simulink model "Simulation"  (R2023b)
settings: Solver=ode4  StartTime=0.0  StopTime=Te  FixedStep=Ts/20  RelTol=1e-3
undefined symbols (not defined in the file): driving, EgoCar1_params, MPC, mv0, targetSpeed, Ts, waypoints, Weights, x0
libraries: drivingscenarioandsensors x7, robotcorelib x2, mpclib x1, trackingutilitieslib x1, sensorinslib x1, drivinglib x1
settings Model: NumberOfSteps=10  SnapshotBufferSize=1000  SnapshotInterval=100  Creator=Victor  LastModifiedBy=Administrator
settings SolverCC: ZeroCrossAlgorithm=Adaptive
settings DebuggingCC: IgnoredZcDiagnostic=none
settings RTWCC: Toolchain=MinGW64 | CMake/gmake (64-bit Windows)  BuildConfiguration=Release

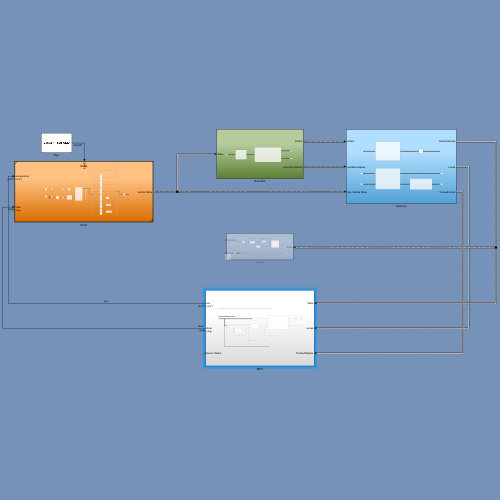
[thumbnail: Simulink's stored preview of the top-level diagram]
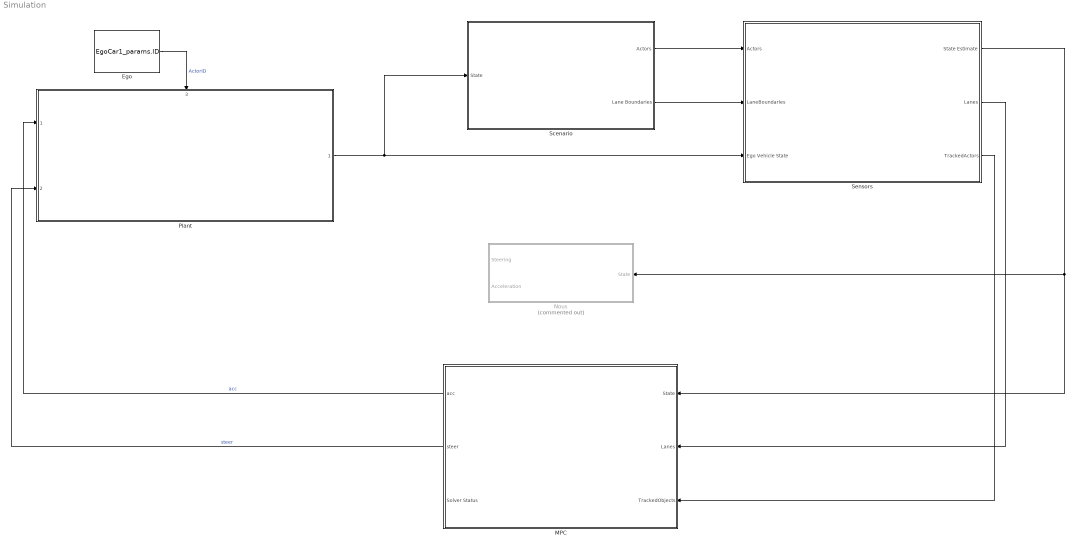
== system Simulation ==
  Ego : Constant  Value=EgoCar1_params.ID
  MPC : Subsystem
  Nous : Subsystem  Commented=on  TreatAsAtomicUnit=on  SystemSampleTime=Ts
  Plant : Subsystem  TreatAsAtomicUnit=on  ReferencedSubsystem=Soma
      settings: MinAlgLoopOccurrences=on  PortSchema="{\"entries\":[{\"content\":{\"sides\":[{\"content\":{\"connectorIds\":[\"In1\",\"In2\"]},\"type\":\"ConnectorPlacement.EquallySpacedRectSide\",\"uuid\":\"82aec969-d257-4f7e-b4fb-71e676d562f3\"},{\"content\":{\"connectorIds\":[\"Out1\"],\"side\":\"RIGHT\"},\"type\":\"ConnectorPlacement.EquallySpacedRectSide\",\"uuid\":\"f71f46c3-49a0-4a72-a46c-a54026d0f764\"},{\"content\":{\"connectorIds\":[\"In3\"],\"side\":\"TOP\"},\"type\":\"ConnectorPlacement.EquallySpacedRectSide\",\"uuid\":\"bd658373-d3b1-4890-887d-293a026755f3\"}]},\"type\":\"ConnectorPlacement.EquallySpacedConnector\",\"uuid\":\"711f2f1f-5cb1-45fa-aff1-e378691897a1\"}],\"packageUris\":[\"http://schema.mathworks.com/mf0/Connector/R2020b\"],\"version\":\"1.0\"}"
  Scenario : Subsystem  SystemSampleTime=Ts
  Sensors : Subsystem
  wires:
  Sensors/1(State Estimate) -> Nous/1(State), MPC/1(State)
  MPC/1(acc) -> Plant/1  "acc"
  MPC/2(steer) -> Plant/2  "steer"
  Ego/1 -> Plant/3  "ActorID"
  Plant/1 -> Scenario/1(State), Sensors/3(Ego Vehicle State)
  Scenario/1(Actors) -> Sensors/1(Actors)
  Scenario/2(Lane Boundaries) -> Sensors/2(LaneBoundaries)
  Sensors/2(Lanes) -> MPC/2(Lanes)
  Sensors/3(TrackedActors) -> MPC/3(TrackedObjects)

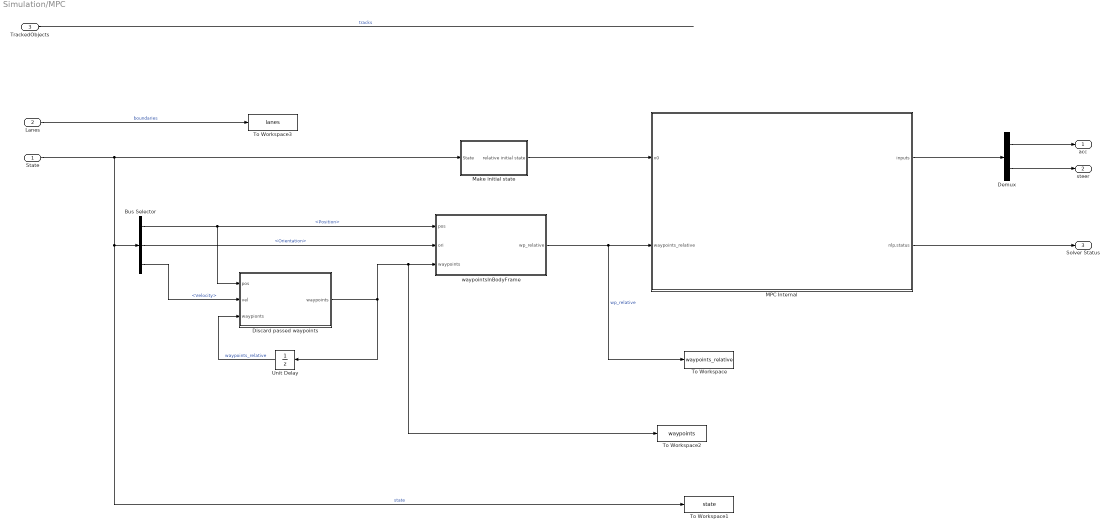
== system Simulation/MPC ==
  State : Inport  OutDataTypeStr=Bus: BusEgoVehicleState  SampleTime=Ts
  Lanes : Inport  Port=2  SampleTime=Ts
  TrackedObjects : Inport  Port=3  SampleTime=Ts
  Bus Selector : BusSelector  OutputSignals=Position,Orientation,Velocity
  Demux : Demux  Outputs=2
  Discard passed waypoints : MATLAB Function  TreatAsAtomicUnit=on
  MPC Internal : Subsystem
  Make initial state : Subsystem
  To Workspace : ToWorkspace  VariableName=waypoints_relative  SaveFormat=Timeseries  SampleTime=-1
  To Workspace1 : ToWorkspace  VariableName=state  SaveFormat=Timeseries  SampleTime=-1
  To Workspace2 : ToWorkspace  VariableName=waypoints  SaveFormat=Timeseries  SampleTime=-1
  To Workspace3 : ToWorkspace  VariableName=lanes  SaveFormat=Timeseries  SampleTime=-1
  Unit Delay : UnitDelay  InitialCondition=waypoints  SampleTime=Ts  HasFrameUpgradeWarning=on
  waypointsInBodyFrame : MATLAB Function  TreatAsAtomicUnit=on
  acc : Outport  Unit=m/s^2  PortDimensions=1  SampleTime=Ts
  steer : Outport  Port=2  Unit=deg  PortDimensions=1  SampleTime=Ts
  Solver Status : Outport  Port=3
  wires:
  State/1 -> Make initial state/1(State), To Workspace1/1, Bus Selector/1  "state"
  Bus Selector/1 -> Discard passed waypoints/1(pos), waypointsInBodyFrame/1(pos)  "<Position>"
  Bus Selector/3 -> Discard passed waypoints/2(vel)  "<Velocity>"
  TrackedObjects/1 -> ?  "tracks"
  waypointsInBodyFrame/1(wp_relative) -> To Workspace/1, MPC Internal/2(waypoints_relative)  "wp_relative"
  Lanes/1 -> To Workspace3/1  "boundaries"
  Demux/1 -> acc/1
  Demux/2 -> steer/1
  MPC Internal/2(nlp.status) -> Solver Status/1
  MPC Internal/1(inputs) -> Demux/1
  Make initial state/1(relative initial state) -> MPC Internal/1(x0)
  Discard passed waypoints/1(waypoints) -> Unit Delay/1, To Workspace2/1, waypointsInBodyFrame/3(waypoints)
  Bus Selector/2 -> waypointsInBodyFrame/2(ori)  "<Orientation>"
  Unit Delay/1 -> Discard passed waypoints/3(waypionts)  "waypoints_relative"

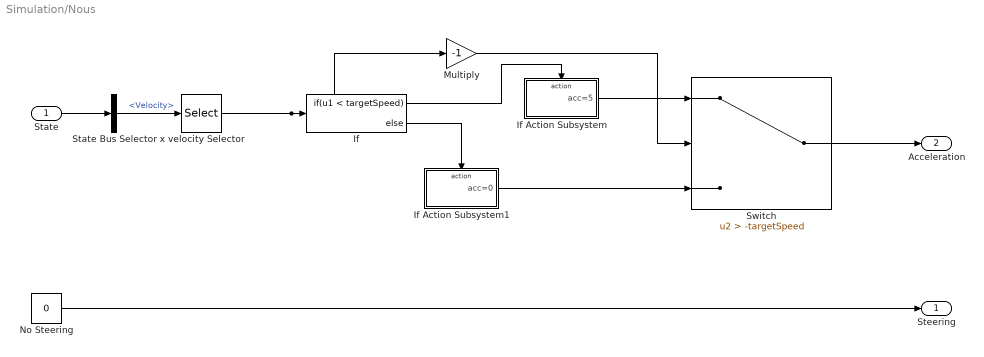
== system Simulation/Nous ==
  State : Inport  SampleTime=Ts
  If : If  IfExpression=u1 < targetSpeed
  If Action Subsystem : Subsystem  TreatAsAtomicUnit=on
  If Action Subsystem1 : Subsystem  TreatAsAtomicUnit=on
  Multiply : Gain  Gain=-1
  No Steering : Constant  Value=0  SampleTime=Ts
  State Bus Selector : BusSelector  OutputSignals=Velocity
  Switch : Switch  Criteria=u2 > Threshold  Threshold=-targetSpeed  SaturateOnIntegerOverflow=off  InputSameDT=off
  x velocity Selector : Selector  InputPortWidth=3  IndexOptions=Index vector (dialog)  Indices=[1]  OutputSizes=1
  Steering : Outport  Unit=deg  SampleTime=Ts
  Acceleration : Outport  Port=2  Unit=m/s^2  SampleTime=Ts
  wires:
  Switch/1 -> Acceleration/1
  If Action Subsystem/1(acc=5) -> Switch/1
  If/1 -> If Action Subsystem/Action
  State/1 -> State Bus Selector/1
  x velocity Selector/1 -> Multiply/1, If/1
  If Action Subsystem1/1(acc=0) -> Switch/3
  No Steering/1 -> Steering/1
  Multiply/1 -> Switch/2
  State Bus Selector/1 -> x velocity Selector/1  "<Velocity>"
  If/2 -> If Action Subsystem1/Action

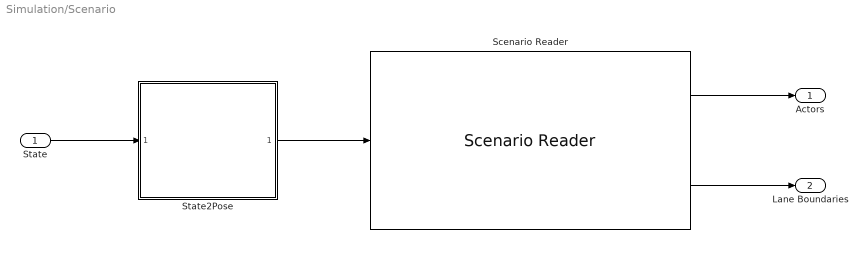
== system Simulation/Scenario ==
  State : Inport
  " State2Pose" : Subsystem  TreatAsAtomicUnit=on  ReferencedSubsystem=State2Pose
  Scenario Reader : drivingscenarioandsensors/Scenario Reader  ScenarioSource=From file  ScenarioFileName=C:\Users\Administrator\Projects\RNNMPC\Scenarios\StraightRoad_Challenge.mat  ScenarioVariableName=Scenario  OutputCoordinateSystem=Vehicle coordinates  EgoVehicleSource=Input port  EgoVehicleActorID=1  OrientVehiclesOnRoad=on  OutputEgoVehiclePose=off  OutputEgoVehicleState=on  SampleTime=Ts  LaneBoundaryOutput=All lane boundaries  LaneBoundaryDistance=linspace(0, 50, 51)  LaneBoundaryLocation=Center of lane markings  BusNameSource=Auto  BusName=BusActors  BusNumActorsSource=Scenario  BusNumActors=32  BusName2Source=Auto  BusName2=BusLaneBoundaries  BusNumLaneBoundariesSource=Scenario  BusNumLaneBoundaries=10  BusName3Source=Auto  BusName3=BusEgoActor  BusName4Source=Auto  BusName4=BusEgoState  ShowCoordinateLabels=on  SimulateUsing=Code generation
  Actors : Outport
  Lane Boundaries : Outport  Port=2
  wires:
  Scenario Reader/1 -> Actors/1
  State/1 -> " State2Pose"/1
  Scenario Reader/2 -> Lane Boundaries/1
  " State2Pose"/1 -> Scenario Reader/1

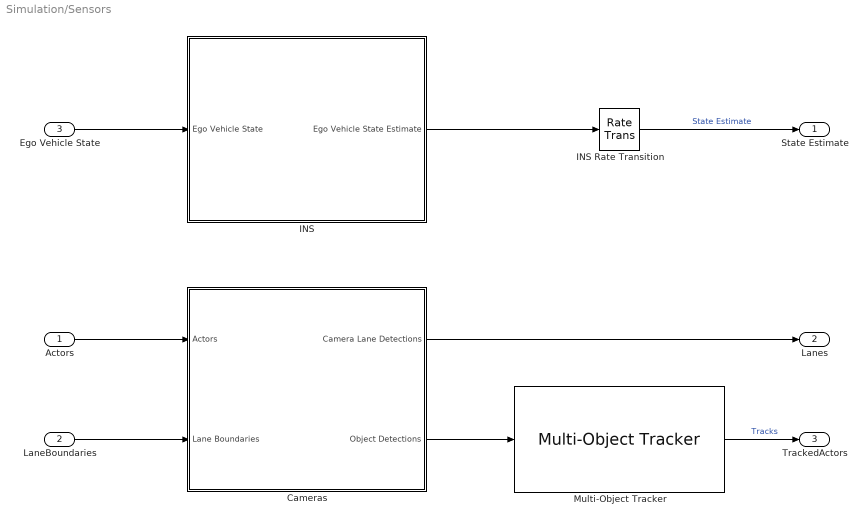
== system Simulation/Sensors ==
  Actors : Inport
  LaneBoundaries : Inport  Port=2
  Ego Vehicle State : Inport  Port=3  OutDataTypeStr=Bus: BusEgoVehicleState
  Cameras : Subsystem
  INS : Subsystem  TreatAsAtomicUnit=on  SystemSampleTime=Ts
  INS Rate Transition : RateTransition  OutPortSampleTime=Ts
  Multi-Object Tracker : drivinglib/Multi-Object Tracker  TrackerIndex=uint32( 0 )  FilterInitializationFcn=initcvekf  AssignmentThreshold=50  ConfirmationThreshold=[ 2, 3 ]  DeletionThreshold=[5,5]  MaxNumTracks=6  MaxNumSensors=8  OOSMHandling=Terminate  StateParametersSimulink=struct  HasStateParametersInput=off  TimeInputSource=Auto  HasCostMatrixInput=off  HasDetectableTrackIDsInput=off  BusNameSource=Auto  BusName=BusMultiObjectTracker1  TentativeTracksOutputPort=off  AllTracksOutputPort=off  SimulateUsing=Interpreted execution
  State Estimate : Outport
  Lanes : Outport  Port=2  SampleTime=Ts
  TrackedActors : Outport  Port=3  SampleTime=Ts
  wires:
  Ego Vehicle State/1 -> INS/1(Ego Vehicle State)
  INS Rate Transition/1 -> State Estimate/1  "State Estimate"
  INS/1(Ego Vehicle State Estimate) -> INS Rate Transition/1
  Multi-Object Tracker/1 -> TrackedActors/1  "Tracks"
  Actors/1 -> Cameras/1(Actors)
  LaneBoundaries/1 -> Cameras/2(Lane Boundaries)
  Cameras/1(Camera Lane Detections) -> Lanes/1
  Cameras/2(Object Detections) -> Multi-Object Tracker/1

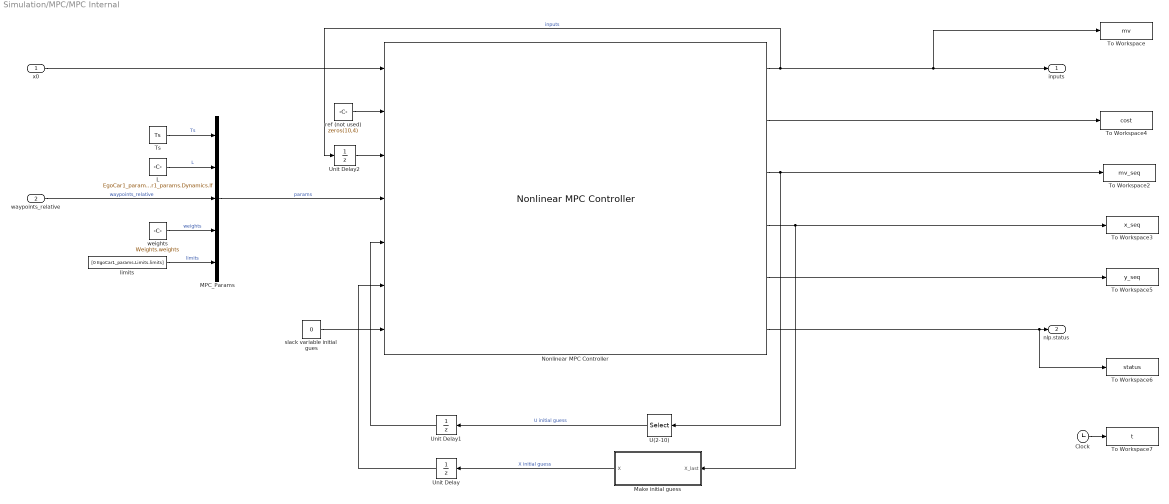
== system Simulation/MPC/MPC Internal ==
  x0 : Inport
  waypoints_relative : Inport  Port=2
  Clock : Clock
  L : Constant  Value=EgoCar1_params.Dynamics.lr+EgoCar1_params.Dynamics.lf  SampleTime=Ts
  MPC_Params : BusCreator  Inputs=5  OutDataTypeStr=Bus: BusParams  NonVirtualBus=on
      settings: InheritFromInputs=off
  Make initial guess : MATLAB Function  TreatAsAtomicUnit=on
  Nonlinear MPC Controller : mpclib/Nonlinear MPC Controller  nlmpcobj=MPC  UseObjectTs=on  UseMEX=off  mexname=nlmpc_MEX  md_enabled=off  mvtarget_enabled=off  param_enabled=on  cost_enabled=on  mvseq_enabled=on  stateseq_enabled=on  ovseq_enabled=on  slack_enabled=off  status_enabled=on  ov_min=off  ov_max=off  mv_min=off  mv_max=off  mvrate_min=off  mvrate_max=off  state_min=off  state_max=off  ov_weight=off  mv_weight=off  mvrate_weight=off  ecr_weight=off  nlp_initialize=on
  To Workspace : ToWorkspace  VariableName=mv  SaveFormat=Timeseries  SampleTime=-1
  To Workspace2 : ToWorkspace  VariableName=mv_seq  SaveFormat=Timeseries  SampleTime=-1
  To Workspace3 : ToWorkspace  VariableName=x_seq  SaveFormat=Timeseries  SampleTime=-1
  To Workspace4 : ToWorkspace  VariableName=cost  SaveFormat=Timeseries  SampleTime=-1
  To Workspace5 : ToWorkspace  VariableName=y_seq  SaveFormat=Timeseries  SampleTime=-1
  To Workspace6 : ToWorkspace  VariableName=status  SaveFormat=Timeseries  SampleTime=-1
  To Workspace7 : ToWorkspace  VariableName=t  SaveFormat=Timeseries  SampleTime=-1
  Ts : Constant  Value=Ts  SampleTime=Ts
  U(2-10) : Selector  NumberOfDimensions=2  InputPortWidth=3  IndexOptions=Index vector (dialog),Index vector (dialog)  Indices=[2:MPC.PredictionHorizon+1],[1:2]  OutputSizes=1,1
  Unit Delay : UnitDelay  InitialCondition=repmat(x0',10,1)  SampleTime=Ts  HasFrameUpgradeWarning=on
  Unit Delay1 : UnitDelay  InitialCondition=repmat(mv0',10,1)  SampleTime=Ts  HasFrameUpgradeWarning=on
  Unit Delay2 : UnitDelay  SampleTime=Ts  HasFrameUpgradeWarning=on
  limits : FromWorkspace  VariableName=[0 EgoCar1_params.Limits.limits]  SampleTime=Ts  Interpolate=off  OutputAfterFinalValue=Holding final value
  ref (not used) : Constant  Value=zeros(10,4)
  slack variable initial gues : Constant  Value=0
  weights : Constant  Value=Weights.weights  SampleTime=Ts
  inputs : Outport
  nlp.status : Outport  Port=2
  wires:
  Nonlinear MPC Controller/5 -> To Workspace5/1
  Nonlinear MPC Controller/1 -> To Workspace/1, inputs/1, Unit Delay2/1  "inputs"
  Nonlinear MPC Controller/6 -> To Workspace6/1, nlp.status/1
  Unit Delay1/1 -> Nonlinear MPC Controller/5
  slack variable initial gues/1 -> Nonlinear MPC Controller/7
  ref (not used)/1 -> Nonlinear MPC Controller/2
  Nonlinear MPC Controller/3 -> To Workspace2/1, U(2-10)/1
  U(2-10)/1 -> Unit Delay1/1  "U initial guess"
  Unit Delay/1 -> Nonlinear MPC Controller/6
  Unit Delay2/1 -> Nonlinear MPC Controller/3
  Nonlinear MPC Controller/2 -> To Workspace4/1
  waypoints_relative/1 -> MPC_Params/3  "waypoints_relative"
  x0/1 -> Nonlinear MPC Controller/1
  L/1 -> MPC_Params/2  "L"
  Ts/1 -> MPC_Params/1  "Ts"
  weights/1 -> MPC_Params/4  "weights"
  MPC_Params/1 -> Nonlinear MPC Controller/4  "params"
  limits/1 -> MPC_Params/5  "limits"
  Make initial guess/1(X) -> Unit Delay/1  "X initial guess"
  Nonlinear MPC Controller/4 -> Make initial guess/1(X_last), To Workspace3/1
  Clock/1 -> To Workspace7/1

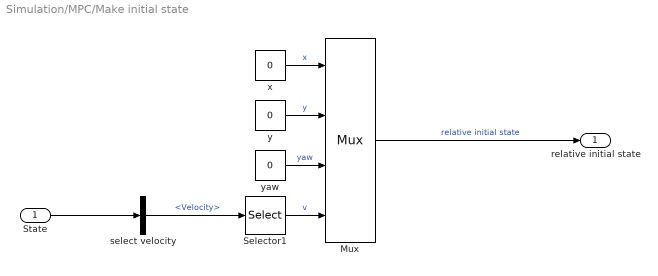
== system Simulation/MPC/Make initial state ==
  State : Inport
  Mux : Mux
      settings: DisplayOption=signals
  Selector1 : Selector  InputPortWidth=3  IndexOptions=Index vector (dialog)  Indices=1  OutputSizes=1
  select velocity : BusSelector  OutputSignals=Velocity
  x : Constant  Value=0
  y : Constant  Value=0
  yaw : Constant  Value=0
  relative initial state : Outport
  wires:
  y/1 -> Mux/2  "y"
  Mux/1 -> relative initial state/1  "relative initial state"
  x/1 -> Mux/1  "x"
  yaw/1 -> Mux/3  "yaw"
  Selector1/1 -> Mux/4  "v"
  select velocity/1 -> Selector1/1  "<Velocity>"
  State/1 -> select velocity/1

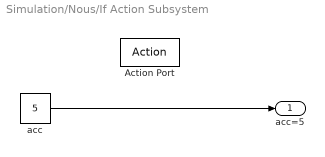
== system Simulation/Nous/If Action Subsystem ==
  Action Port : ActionPort  ActionPortLabel=if(u1 < targetSpeed)
  acc : Constant  Value=5
  acc=5 : Outport
  wires:
  acc/1 -> acc=5/1

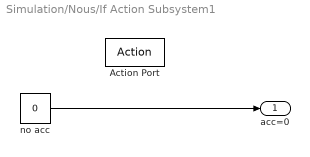
== system Simulation/Nous/If Action Subsystem1 ==
  Action Port : ActionPort  ActionPortLabel=else
  no acc : Constant  Value=0
  acc=0 : Outport
  wires:
  no acc/1 -> acc=0/1

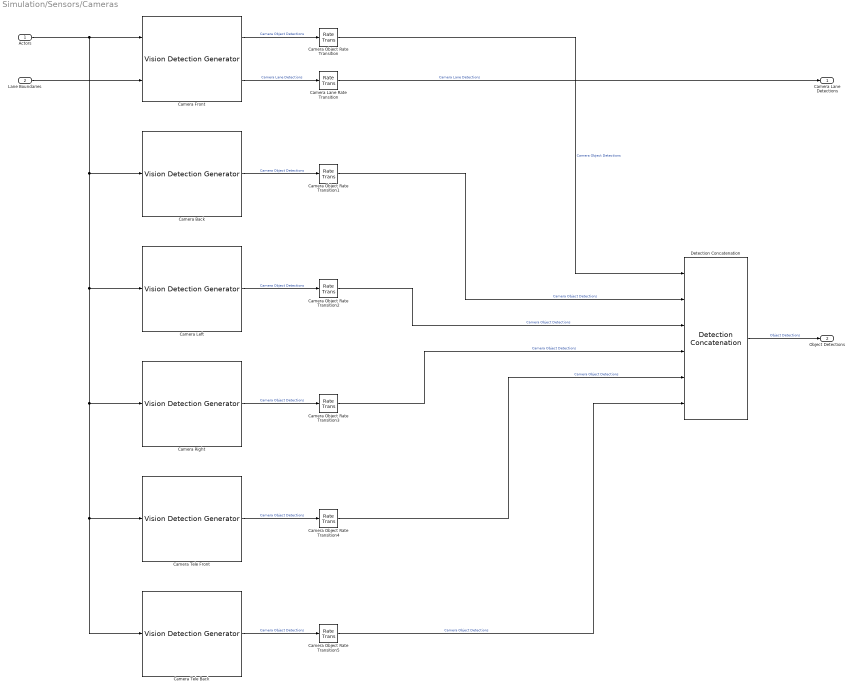
== system Simulation/Sensors/Cameras ==
  Actors : Inport
  Lane Boundaries : Inport  Port=2
  Camera Back : drivingscenarioandsensors/Vision Detection Generator  SensorIndex=3  DetectorOutput=Objects only  UpdateInterval=Ts  LaneUpdateInterval=Ts  SensorLocation=[ 1.9, 0 ]  Height=1.1  Yaw=EgoCar1_params.Sensors.cameras(2).Direction  Pitch=1  Roll=0  BusNameSource=Auto  BusName=BusObjectDetections  BusName2Source=Auto  BusName2=BusLaneDetections  MaxNumDetectionsSource=Property  MaxNumDetections=6  MaxNumLanesSource=Property  MaxNumLanes=30  DetectionCoordinates=Ego Cartesian  SimulateUsing=Code generation  MaxRange=EgoCar1_params.Sensors.cameras(2).Range_Max  BoundingBoxAccuracy=5  ProcessNoiseIntensity=5  MaxSpeed=100  MaxAllowedOcclusion=0.5  MinObjectImageSize=[ 15, 15 ]  DetectionProbability=0.9  FalsePositivesPerImage=0  MinLaneImageSize=[ 20, 3 ]  LaneBoundaryAccuracy=3  HasNoise=off  InitialSeedSource=Repeatable  InitialSeed=0  UsedSeed=driving.internal.SimulinkUtilities.seedManager(gcb)  ActorProfilesSource=From Scenario Reader block  ActorProfilesParameters=driving.internal.ActorProfilesParameters  ActorProfilesExpression=struct( 'ClassID', 0, 'Length', 4.7, 'Width', 1.8, 'Height', 1.4, 'OriginOffset', [ -1.35, 0, 0 ] )  Intrinsics=driving.internal.cameraIntrinsics(FocalLength=[ EgoCar1_params.Sensors.cameras(2).FocalLength_X, EgoCar1_params.Sensors.cameras(2).FocalLength_Y],PrincipalPoint=[ EgoCar1_params.Sensors.cameras(2).OpticalCenter_X, EgoCar1_params.Sensors.cameras(2).OpticalCenter_Y],ImageSize=[ EgoCar1_params.Sensors.cameras(2).Image_Height, EgoCar1_params.Sensors.cameras(2).Image_Width])
  Camera Front : drivingscenarioandsensors/Vision Detection Generator  SensorIndex=2  DetectorOutput=Lanes and objects  UpdateInterval=Ts  LaneUpdateInterval=Ts  SensorLocation=[ 1.9, 0 ]  Height=1.1  Yaw=EgoCar1_params.Sensors.cameras(1).Direction  Pitch=1  Roll=0  BusNameSource=Auto  BusName=BusObjectDetections  BusName2Source=Auto  BusName2=BusLaneDetections  MaxNumDetectionsSource=Property  MaxNumDetections=6  MaxNumLanesSource=Property  MaxNumLanes=12  DetectionCoordinates=Ego Cartesian  SimulateUsing=Code generation  MaxRange=EgoCar1_params.Sensors.cameras(1).Range_Max  BoundingBoxAccuracy=5  ProcessNoiseIntensity=5  MaxSpeed=100  MaxAllowedOcclusion=0.5  MinObjectImageSize=[ 15, 15 ]  DetectionProbability=0.9  FalsePositivesPerImage=0  MinLaneImageSize=[10, 3]  LaneBoundaryAccuracy=3  HasNoise=off  InitialSeedSource=Repeatable  InitialSeed=0  UsedSeed=driving.internal.SimulinkUtilities.seedManager(gcb)  ActorProfilesSource=From Scenario Reader block  ActorProfilesParameters=driving.internal.ActorProfilesParameters  ActorProfilesExpression=struct( 'ClassID', 0, 'Length', 4.7, 'Width', 1.8, 'Height', 1.4, 'OriginOffset', [ -1.35, 0, 0 ] )  Intrinsics=driving.internal.cameraIntrinsics(FocalLength=[ EgoCar1_params.Sensors.cameras(1).FocalLength_X, EgoCar1_params.Sensors.cameras(1).FocalLength_Y],PrincipalPoint=[ EgoCar1_params.Sensors.cameras(1).OpticalCenter_X, EgoCar1_params.Sensors.cameras(1).OpticalCenter_Y],ImageSize=[ EgoCar1_params.Sensors.cameras(1).Image_Height, EgoCar1_params.Sensors.cameras(1).Image_Width])
  Camera Lane Rate Transition : RateTransition  OutPortSampleTime=Ts
  Camera Left : drivingscenarioandsensors/Vision Detection Generator  SensorIndex=4  DetectorOutput=Objects only  UpdateInterval=Ts  LaneUpdateInterval=Ts  SensorLocation=[ 1.9, 0 ]  Height=1.1  Yaw=EgoCar1_params.Sensors.cameras(3).Direction  Pitch=1  Roll=0  BusNameSource=Auto  BusName=BusObjectDetections  BusName2Source=Auto  BusName2=BusLaneDetections  MaxNumDetectionsSource=Property  MaxNumDetections=6  MaxNumLanesSource=Property  MaxNumLanes=30  DetectionCoordinates=Ego Cartesian  SimulateUsing=Code generation  MaxRange=EgoCar1_params.Sensors.cameras(3).Range_Max  BoundingBoxAccuracy=5  ProcessNoiseIntensity=5  MaxSpeed=100  MaxAllowedOcclusion=0.5  MinObjectImageSize=[ 15, 15 ]  DetectionProbability=0.9  FalsePositivesPerImage=0  MinLaneImageSize=[ 20, 3 ]  LaneBoundaryAccuracy=3  HasNoise=off  InitialSeedSource=Repeatable  InitialSeed=0  UsedSeed=driving.internal.SimulinkUtilities.seedManager(gcb)  ActorProfilesSource=From Scenario Reader block  ActorProfilesParameters=driving.internal.ActorProfilesParameters  ActorProfilesExpression=struct( 'ClassID', 0, 'Length', 4.7, 'Width', 1.8, 'Height', 1.4, 'OriginOffset', [ -1.35, 0, 0 ] )  Intrinsics=driving.internal.cameraIntrinsics(FocalLength=[ EgoCar1_params.Sensors.cameras(3).FocalLength_X, EgoCar1_params.Sensors.cameras(3).FocalLength_Y],PrincipalPoint=[ EgoCar1_params.Sensors.cameras(3).OpticalCenter_X, EgoCar1_params.Sensors.cameras(3).OpticalCenter_Y],ImageSize=[ EgoCar1_params.Sensors.cameras(3).Image_Height, EgoCar1_params.Sensors.cameras(3).Image_Width])
  Camera Object Rate Transition{,1..5} (6 alike) : RateTransition  OutPortSampleTime=Ts
  Camera Right : drivingscenarioandsensors/Vision Detection Generator  SensorIndex=5  DetectorOutput=Objects only  UpdateInterval=Ts  LaneUpdateInterval=Ts  SensorLocation=[ 1.9, 0 ]  Height=1.1  Yaw=EgoCar1_params.Sensors.cameras(4).Direction  Pitch=1  Roll=0  BusNameSource=Auto  BusName=BusObjectDetections  BusName2Source=Auto  BusName2=BusLaneDetections  MaxNumDetectionsSource=Property  MaxNumDetections=6  MaxNumLanesSource=Property  MaxNumLanes=30  DetectionCoordinates=Ego Cartesian  SimulateUsing=Code generation  MaxRange=EgoCar1_params.Sensors.cameras(4).Range_Max  BoundingBoxAccuracy=5  ProcessNoiseIntensity=5  MaxSpeed=100  MaxAllowedOcclusion=0.5  MinObjectImageSize=[ 15, 15 ]  DetectionProbability=0.9  FalsePositivesPerImage=0  MinLaneImageSize=[ 20, 3 ]  LaneBoundaryAccuracy=3  HasNoise=off  InitialSeedSource=Repeatable  InitialSeed=0  UsedSeed=driving.internal.SimulinkUtilities.seedManager(gcb)  ActorProfilesSource=From Scenario Reader block  ActorProfilesParameters=driving.internal.ActorProfilesParameters  ActorProfilesExpression=struct( 'ClassID', 0, 'Length', 4.7, 'Width', 1.8, 'Height', 1.4, 'OriginOffset', [ -1.35, 0, 0 ] )  Intrinsics=driving.internal.cameraIntrinsics(FocalLength=[ EgoCar1_params.Sensors.cameras(4).FocalLength_X, EgoCar1_params.Sensors.cameras(4).FocalLength_Y],PrincipalPoint=[ EgoCar1_params.Sensors.cameras(4).OpticalCenter_X, EgoCar1_params.Sensors.cameras(4).OpticalCenter_Y],ImageSize=[ EgoCar1_params.Sensors.cameras(4).Image_Height, EgoCar1_params.Sensors.cameras(4).Image_Width])
  Camera Tele Back : drivingscenarioandsensors/Vision Detection Generator  SensorIndex=7  DetectorOutput=Objects only  UpdateInterval=Ts  LaneUpdateInterval=Ts  SensorLocation=[ 1.9, 0 ]  Height=1.1  Yaw=EgoCar1_params.Sensors.cameras(6).Direction  Pitch=1  Roll=0  BusNameSource=Auto  BusName=BusObjectDetections  BusName2Source=Auto  BusName2=BusLaneDetections  MaxNumDetectionsSource=Property  MaxNumDetections=6  MaxNumLanesSource=Property  MaxNumLanes=30  DetectionCoordinates=Ego Cartesian  SimulateUsing=Code generation  MaxRange=EgoCar1_params.Sensors.cameras(6).Range_Max  BoundingBoxAccuracy=5  ProcessNoiseIntensity=5  MaxSpeed=100  MaxAllowedOcclusion=0.5  MinObjectImageSize=[ 15, 15 ]  DetectionProbability=0.9  FalsePositivesPerImage=0  MinLaneImageSize=[10, 3]  LaneBoundaryAccuracy=3  HasNoise=off  InitialSeedSource=Repeatable  InitialSeed=0  UsedSeed=driving.internal.SimulinkUtilities.seedManager(gcb)  ActorProfilesSource=From Scenario Reader block  ActorProfilesParameters=driving.internal.ActorProfilesParameters  ActorProfilesExpression=struct( 'ClassID', 0, 'Length', 4.7, 'Width', 1.8, 'Height', 1.4, 'OriginOffset', [ -1.35, 0, 0 ] )  Intrinsics=driving.internal.cameraIntrinsics(FocalLength=[ EgoCar1_params.Sensors.cameras(6).FocalLength_X, EgoCar1_params.Sensors.cameras(6).FocalLength_Y],ImageSize=[ EgoCar1_params.Sensors.cameras(6).Image_Height, EgoCar1_params.Sensors.cameras(6).Image_Width],PrincipalPoint=[ EgoCar1_params.Sensors.cameras(6).OpticalCenter_X, EgoCar1_params.Sensors.cameras(6).OpticalCenter_Y])
  Camera Tele Front : drivingscenarioandsensors/Vision Detection Generator  SensorIndex=6  DetectorOutput=Objects only  UpdateInterval=Ts  LaneUpdateInterval=Ts  SensorLocation=[ 1.9, 0 ]  Height=1.1  Yaw=EgoCar1_params.Sensors.cameras(5).Direction  Pitch=1  Roll=0  BusNameSource=Auto  BusName=BusObjectDetections  BusName2Source=Auto  BusName2=BusLaneDetections  MaxNumDetectionsSource=Property  MaxNumDetections=6  MaxNumLanesSource=Property  MaxNumLanes=30  DetectionCoordinates=Ego Cartesian  SimulateUsing=Code generation  MaxRange=EgoCar1_params.Sensors.cameras(5).Range_Max  BoundingBoxAccuracy=5  ProcessNoiseIntensity=5  MaxSpeed=100  MaxAllowedOcclusion=0.5  MinObjectImageSize=[ 15, 15 ]  DetectionProbability=0.9  FalsePositivesPerImage=0  MinLaneImageSize=[10, 3]  LaneBoundaryAccuracy=3  HasNoise=off  InitialSeedSource=Repeatable  InitialSeed=0  UsedSeed=driving.internal.SimulinkUtilities.seedManager(gcb)  ActorProfilesSource=From Scenario Reader block  ActorProfilesParameters=driving.internal.ActorProfilesParameters  ActorProfilesExpression=struct( 'ClassID', 0, 'Length', 4.7, 'Width', 1.8, 'Height', 1.4, 'OriginOffset', [ -1.35, 0, 0 ] )  Intrinsics=driving.internal.cameraIntrinsics(FocalLength=[ EgoCar1_params.Sensors.cameras(5).FocalLength_X, EgoCar1_params.Sensors.cameras(5).FocalLength_Y],ImageSize=[ EgoCar1_params.Sensors.cameras(5).Image_Height, EgoCar1_params.Sensors.cameras(5).Image_Width],PrincipalPoint=[ EgoCar1_params.Sensors.cameras(5).OpticalCenter_X, EgoCar1_params.Sensors.cameras(5).OpticalCenter_Y])
  Detection Concatenation : trackingutilitieslib/Detection Concatenation  NumInputs=6  BusNameSource=Auto  BusName=BusDetectionConcatenation1  SimulateUsing=Interpreted execution
  Camera Lane Detections : Outport
  Object Detections : Outport  Port=2
  wires:
  Camera Front/1 -> Camera Object Rate Transition/1  "Camera Object Detections"
  Camera Left/1 -> Camera Object Rate Transition2/1  "Camera Object Detections"
  Camera Lane Rate Transition/1 -> Camera Lane Detections/1  "Camera Lane Detections"
  Camera Right/1 -> Camera Object Rate Transition3/1  "Camera Object Detections"
  Lane Boundaries/1 -> Camera Front/2
  Camera Object Rate Transition/1 -> Detection Concatenation/1  "Camera Object Detections"
  Camera Object Rate Transition1/1 -> Detection Concatenation/2  "Camera Object Detections"
  Detection Concatenation/1 -> Object Detections/1  "Object Detections"
  Camera Front/2 -> Camera Lane Rate Transition/1  "Camera Lane Detections"
  Camera Object Rate Transition3/1 -> Detection Concatenation/4  "Camera Object Detections"
  Camera Object Rate Transition2/1 -> Detection Concatenation/3  "Camera Object Detections"
  Actors/1 -> Camera Tele Back/1, Camera Tele Front/1, Camera Right/1, Camera Left/1, Camera Back/1, Camera Front/1
  Camera Back/1 -> Camera Object Rate Transition1/1  "Camera Object Detections"
  Camera Tele Front/1 -> Camera Object Rate Transition4/1  "Camera Object Detections"
  Camera Object Rate Transition4/1 -> Detection Concatenation/5  "Camera Object Detections"
  Camera Tele Back/1 -> Camera Object Rate Transition5/1  "Camera Object Detections"
  Camera Object Rate Transition5/1 -> Detection Concatenation/6  "Camera Object Detections"

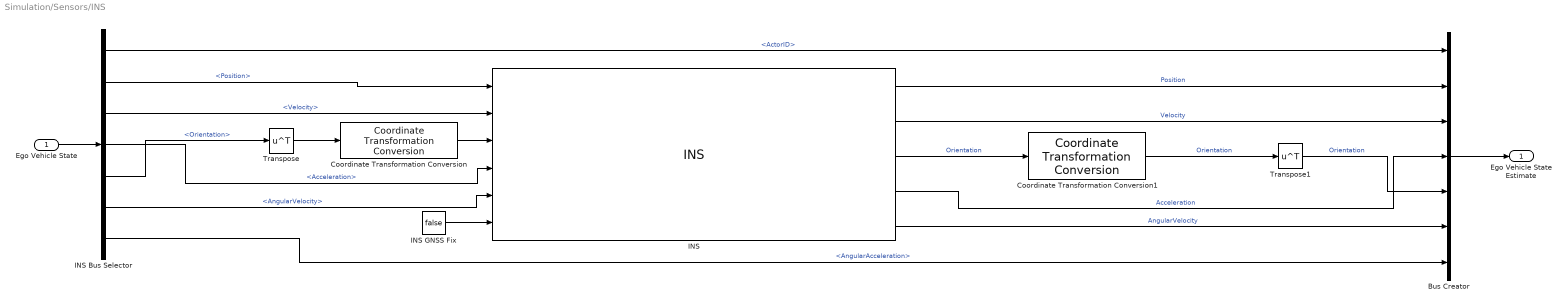
== system Simulation/Sensors/INS ==
  Ego Vehicle State : Inport  OutDataTypeStr=Bus: BusEgoVehicleState
  Bus Creator : BusCreator  Inputs=7  OutDataTypeStr=Bus: BusEgoVehicleState  NonVirtualBus=on
      settings: InheritFromInputs=off
  Coordinate Transformation Conversion : robotcorelib/Coordinate Transformation Conversion  InputRepresentation=Euler Angles  InputEulerSequence=XYZ  ShowTrVecInputPort=on  OutputRepresentation=Rotation Matrix  OutputEulerSequence=ZYX  ShowTrVecOutputPort=on  SimulateUsing=Code generation
      settings: LibrarySourceBlock=navlib/Utilities/Coordinate Transformation Conversion
  Coordinate Transformation Conversion1 : robotcorelib/Coordinate Transformation Conversion  InputRepresentation=Rotation Matrix  InputEulerSequence=ZYX  ShowTrVecInputPort=on  OutputRepresentation=Euler Angles  OutputEulerSequence=XYZ  ShowTrVecOutputPort=on  SimulateUsing=Code generation
      settings: LibrarySourceBlock=navlib/Utilities/Coordinate Transformation Conversion
  INS : sensorinslib/INS  MountingLocation=[0 0 0]  RollAccuracy=EgoCar1_params.Sensors.INS.angleAccuraccy  PitchAccuracy=EgoCar1_params.Sensors.INS.angleAccuraccy  YawAccuracy=EgoCar1_params.Sensors.INS.angleAccuraccy  PositionAccuracy=[EgoCar1_params.Sensors.INS.positionAccuracy EgoCar1_params.Sensors.INS.positionAccuracy EgoCar1_params.Sensors.INS.positionAccuracy]  VelocityAccuracy=EgoCar1_params.Sensors.INS.velocityAccuracy  UseAccelAndAngVel=on  AccelerationAccuracy=0  AngularVelocityAccuracy=0  TimeInput=on  PositionErrorFactor=[0 0 0]  SeedDouble=32  SimulateUsing=Code generation
      settings: LibrarySourceBlock=drivingscenarioandsensors/INS
  INS Bus Selector : BusSelector  OutputSignals=ActorID,Position,Velocity,Acceleration,Orientation,AngularVelocity,AngularAcceleration
  INS GNSS Fix : Constant  Value=false
  Transpose : Math  Operator=transpose
  Transpose1 : Math  Operator=transpose
  Ego Vehicle State Estimate : Outport  OutDataTypeStr=Bus: BusEgoVehicleState
  wires:
  Ego Vehicle State/1 -> INS Bus Selector/1
  INS/2 -> Bus Creator/3  "Velocity"
  Transpose1/1 -> Bus Creator/5  "Orientation"
  INS Bus Selector/3 -> INS/2  "<Velocity>"
  INS/1 -> Bus Creator/2  "Position"
  INS/4 -> Bus Creator/4  "Acceleration"
  Bus Creator/1 -> Ego Vehicle State Estimate/1
  INS/5 -> Bus Creator/6  "AngularVelocity"
  INS GNSS Fix/1 -> INS/6
  Coordinate Transformation Conversion/1 -> INS/3
  INS/3 -> Coordinate Transformation Conversion1/1  "Orientation"
  INS Bus Selector/2 -> INS/1  "<Position>"
  Transpose/1 -> Coordinate Transformation Conversion/1
  Coordinate Transformation Conversion1/1 -> Transpose1/1  "Orientation"
  INS Bus Selector/6 -> INS/5  "<AngularVelocity>"
  INS Bus Selector/1 -> Bus Creator/1  "<ActorID>"
  INS Bus Selector/7 -> Bus Creator/7  "<AngularAcceleration>"
  INS Bus Selector/4 -> INS/4  "<Acceleration>"
  INS Bus Selector/5 -> Transpose/1  "<Orientation>"

== matlab function Simulation/MPC/Discard passed waypoints ==
  data: pos input; waypoints output; vel input; waypionts input
function waypoints = wpts_discard(pos, vel, waypionts)
    waypoints = waypointsTruncation(pos, vel, waypionts);
end

== matlab function Simulation/MPC/MPC Internal/Make initial guess ==
  data: X_last input; X output
function X = makeInitGuess(X_last)
    
    % Discard the state at the previous step
    X=X_last(2:11,:);
    x1=X(1,:);
    
    % Rotation Matrix
    yaw=X(1,3);
    R = [cosd(-yaw), -sind(-yaw); sind(-yaw), cosd(-yaw)];

    for i = 1:size(X,1)
        
        xy=X(i,1:2)';

        % Transformation
        xy=xy-x1(1:2)';
        xy=R * xy;
        X(i,1:2)=xy';

        % Rotation
        X(i,3)=X(i,3)-X(1,3);
    end
end

== matlab function Simulation/MPC/waypointsInBodyFrame ==
  data: pos input; ori input; wp_relative output; waypoints input
function wp_relative = waypointsInBodyFrame(pos, ori, waypoints)
    pos=pos(1:2);
    pos=reshape(pos,2,[]);

    yaw=ori(3);

    wp_relative=NaN(size(waypoints));
    for i=1:size(wp_relative,1)
        wp_relative(i,:) = world2body(pos, yaw, waypoints(i,:)');
    end
end
